simulink model "lock_in_fraser"  (R2021a)
settings: Solver=FixedStepDiscrete  StartTime=0.0  StopTime=Inf  RelTol=1e-3  EnableMultiTasking=on
libraries: dspsrcs4 x2, c2837xDlib x2, dsparch4 x2, c2802xlib x1
settings Model: ExtModeTrigDuration=8  Creator=Fraser Montandon  LastModifiedBy=Fraser Montandon
settings OptimizationCC: DefaultUnderspecifiedDataType=single  EnhancedBackFolding=on  PassReuseOutputArgsAs=Individual arguments  MaxStackSize=1024  OptimizeBlockOrder=speed  DifferentSizesBufferReuse=on  OptimizationCustomize=off  DenormalBehavior=FlushToZero  EfficientTunableParamExpr=on
settings DebuggingCC: ParameterTunabilityLossMsg=error
settings HardwareCC: ProdBitPerChar=16  ProdBitPerInt=16  ProdBitPerPointer=32  ProdBitPerSizeT=32  ProdBitPerPtrDiffT=32  ProdLargestAtomicInteger=Integer  ProdLargestAtomicFloat=None  ProdWordSize=16  ProdLongLongMode=on  ProdHWDeviceType=Texas Instruments->C2000
settings SFSimCC: MATLABDynamicMemAlloc=off
settings RTWCC: SystemTargetFile=ert.tlc  HardwareBoard=TI Delfino F28379D LaunchPad  TemplateMakefile=ert_default_tmf  Toolchain=Texas Instruments Code Composer Studio (C2000)  BuildConfiguration=Faster Runs
settings CodeAppCC: ForceParamTrailComments=on  IgnoreCustomStorageClasses=off  OperatorAnnotations=on  SimulinkDataObjDesc=on  SFDataObjDesc=on  InsertBlockDesc=on
settings ERTTargetCC: CodeReplacementLibrary=TI C28x  ExtModeTransport=3  ExtModeStaticAllocSize=10000

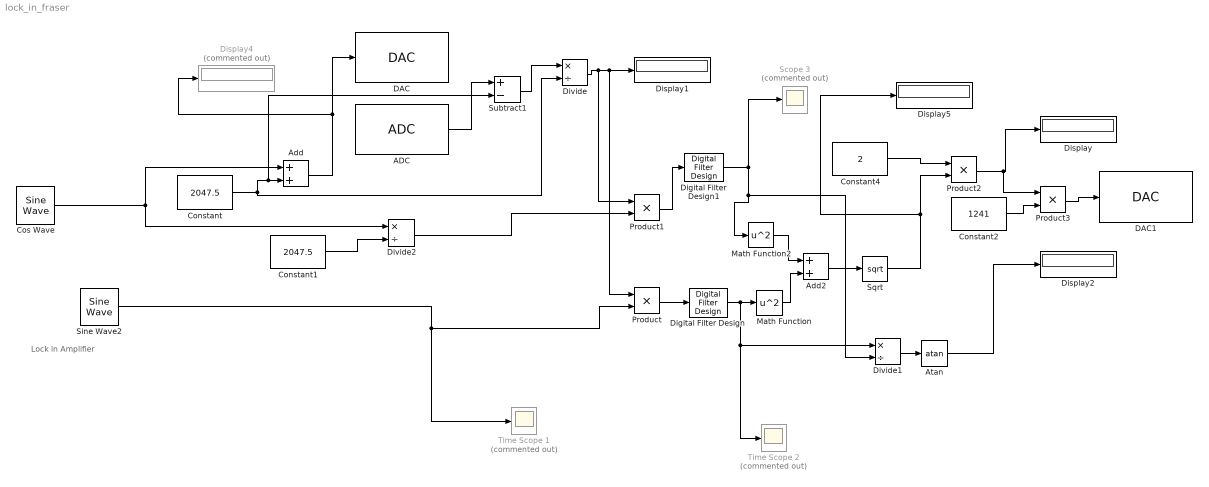
== system lock_in_fraser ==
  note: Lock in Amplifier
  ADC : c2802xlib/ADC  blkParamProc=C2000_Type4  ADCModule=A  samplingMode=Single sample mode  ADCResolution=12-bit (Single-ended input)  useSOC1=SOC0  useSOC2=SOC0_SOC1  SOCAcquisitionWindow=15  SOCTriggerSource=Software  SOCInterruptTrigger=No ADCINT  Ts=1/40000  dType=uint16  postInterrupt=off  interruptSel=ADCINT1  ADCINTContinuous=on  endma=off  chdma=1  conv1=ADCINA0  conv2=ADCINA0 and ADCINB0  conv1_Type4=ADCIN15  conv2_Type4=ADCIN0 and ADCIN1
  Add : Sum
  Add2 : Sum
  Atan : Trigonometry  Operator=atan
  Constant : Constant  Value=2047.5
  Constant1 : Constant  Value=2047.5
  Constant2 : Constant  Value=1241
  Constant4 : Constant  Value=2
  Cos Wave : dspsrcs4/Sine Wave  Amplitude=2047.5  Frequency=2000  Phase=pi/2  SampleMode=Discrete  OutComplex=Real  CompMethod=Table lookup  TableSize=Speed  SampleTime=1/40000  SamplesPerFrame=1  ResetState=Restart at time zero  OutputFrames=off  dataType=double  wordLen=16  udDataType=sfix(16)  fracBitsMode=Best precision  numFracBits=15  OutDataTypeStr=double  LastOutDataTypeStr=double
  DAC : c2837xDlib/DAC  channel=A  saturate=off
      settings: SourceProductBaseCode=TIC2000
  DAC1 : c2837xDlib/DAC  channel=B  saturate=on
      settings: SourceProductBaseCode=TIC2000
  Digital Filter Design : dsparch4/Digital Filter Design  mwdsp_browser_bugfix_var=off
  Digital Filter Design1 : dsparch4/Digital Filter Design  mwdsp_browser_bugfix_var=off
  Display{,1..2,5} (4 alike) : Display
  Display4 : Display  Commented=on
  Divide : Product  Inputs=*/
  Divide1 : Product  Inputs=*/
  Divide2 : Product  Inputs=*/
  Math Function : Math  Operator=square  SaturateOnIntegerOverflow=on
  Math Function2 : Math  Operator=square  SaturateOnIntegerOverflow=on
  Product{,1..3} (4 alike) : Product
  Scope 3 : Scope  Commented=on
  Sine Wave2 : dspsrcs4/Sine Wave  Amplitude=1  Frequency=2000  Phase=0  SampleMode=Discrete  OutComplex=Real  CompMethod=Table lookup  TableSize=Speed  SampleTime=1/40000  SamplesPerFrame=1  ResetState=Restart at time zero  OutputFrames=off  dataType=double  wordLen=16  udDataType=sfix(16)  fracBitsMode=Best precision  numFracBits=15  OutDataTypeStr=double  LastOutDataTypeStr=double
  Sqrt : Sqrt  SaturateOnIntegerOverflow=on
  Subtract1 : Sum  Inputs=+-
  Time Scope 1 : Scope  Commented=on
      settings: Tag=Scope1
  Time Scope 2 : Scope  Commented=on
  wires:
  ADC/1 -> Subtract1/1
  Digital Filter Design1/1 -> Divide1/2, Math Function2/1, Scope 3/1
  Product2/1 -> Product3/1, Display/1
  Sqrt/1 -> Display5/1, Product2/2
  Divide2/1 -> Product1/2
  Constant1/1 -> Divide2/2
  Math Function/1 -> Add2/2
  Product/1 -> Digital Filter Design/1
  Cos Wave/1 -> Divide2/1, Add/1
  Divide1/1 -> Atan/1
  Sine Wave2/1 -> Time Scope 1/1, Product/2
  Add2/1 -> Sqrt/1
  Constant4/1 -> Product2/1
  Divide/1 -> Product1/1, Product/1, Display1/1
  Math Function2/1 -> Add2/1
  Constant/1 -> Subtract1/2, Add/2, Divide/2
  Add/1 -> Display4/1, DAC/1
  Subtract1/1 -> Divide/1
  Digital Filter Design/1 -> Divide1/1, Time Scope 2/1, Math Function/1
  Product1/1 -> Digital Filter Design1/1
  Atan/1 -> Display2/1
  Product3/1 -> DAC1/1
  Constant2/1 -> Product3/2
